simulink model "test_onoff_button_legitbehavior"  (R2022b)
settings: Solver=FixedStepAuto  StartTime=0.0  StopTime=240  FixedStep=0.1  RelTol=1e-3
settings Model: Creator=cristian  LastModifiedBy=cristian
settings ConfigComp: CovEnable=on  RecordCoverage=on  CovModelRefEnable=on

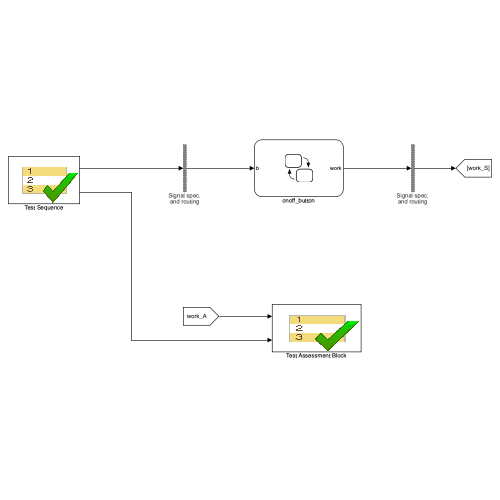
[thumbnail: Simulink's stored preview of the top-level diagram]
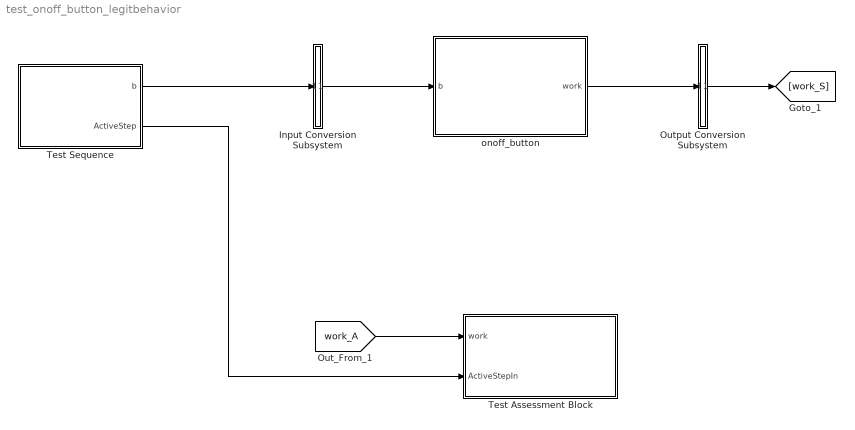
== system test_onoff_button_legitbehavior ==
  Input Conversion Subsystem : Subsystem  Tag=__SLT_ICS__  Description=|
      | Signal spec.
      | and routing
      settings: AttributesFormatString=%<Description>
  Output Conversion Subsystem : Subsystem  Tag=__SLT_OCS__  Description=|
      | Signal spec.
      | and routing
      settings: AttributesFormatString=%<Description>
  Test Assessment Block : Test Sequence  Tag=__SLT_ASMT__  TreatAsAtomicUnit=on
  Test Sequence : Test Sequence  TreatAsAtomicUnit=on
  onoff_button : Stateflow chart  TreatAsAtomicUnit=on
  wires:
  Output Conversion Subsystem/1(Outport_1) -> [work_S]
  Input Conversion Subsystem/1(Outport_1) -> onoff_button/1(b)
  onoff_button/1(work) -> Output Conversion Subsystem/1(Inport_1)
  Test Sequence/1(b) -> Input Conversion Subsystem/1(Inport_1)
  Test Sequence/2(ActiveStep) -> Test Assessment Block/2(ActiveStepIn)
  [work_A] -> Test Assessment Block/1(work)

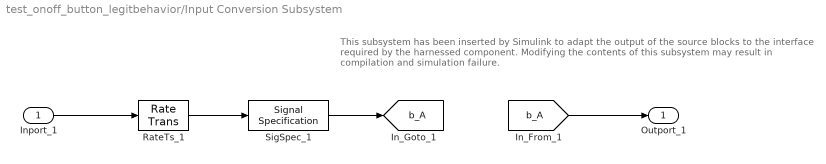
== system test_onoff_button_legitbehavior/Input Conversion Subsystem ==
  note: This subsystem has been inserted by Simulink to adapt the output of the source blocks to the interface required by the harnessed component.
      |  Modifying the contents of this subsystem may result in compilation and simulation failure.
  Inport_1 : Inport
  RateTs_1 : RateTransition  OutPortSampleTime=[-1, 0]
  SigSpec_1 : SignalSpecification  OutDataTypeStr=boolean  Dimensions=[1]  SampleTime=[-1, 0]
  Outport_1 : Outport
  tag scope: b_A=global
  wires:
  [b_A] -> Outport_1/1
  SigSpec_1/1 -> [b_A]
  RateTs_1/1 -> SigSpec_1/1
  Inport_1/1 -> RateTs_1/1

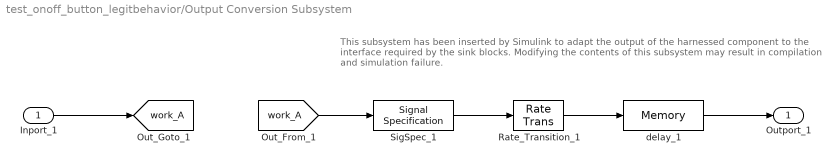
== system test_onoff_button_legitbehavior/Output Conversion Subsystem ==
  note: This subsystem has been inserted by Simulink to adapt the output of the harnessed component to the interface required by the sink blocks.
      |  Modifying the contents of this subsystem may result in compilation and simulation failure.
  Inport_1 : Inport
  Rate_Transition_1 : RateTransition  OutPortSampleTimeOpt=Inherit
  SigSpec_1 : SignalSpecification  OutDataTypeStr=boolean  Dimensions=[1]
  delay_1 : Memory
  Outport_1 : Outport
  tag scope: work_A=global
  wires:
  Inport_1/1 -> [work_A]
  [work_A] -> SigSpec_1/1
  SigSpec_1/1 -> Rate_Transition_1/1
  Rate_Transition_1/1 -> delay_1/1
  delay_1/1 -> Outport_1/1

== stateflow chart test_onoff_button_legitbehavior/Test Assessment Block ==
  state LegitBehavior
    state Run
      state Verify_LB_Init
        verify(work == 0);
      state Verify_LB_Press
        verify(work == 1);
      state Verify_CB_Release
        verify(work == 1);
      state Verify_LB_LongPress
        verify(work == 1);
      state Verify_LB_ReleaseLongPression
        verify(work == 0);
      state Verify_LB_Void
      (junction 388) -> (junction 391) [order 2]
      (junction 387) -> (junction 388) [order 1] : [ActiveStepIn == ActiveStepEnumH2.LB_Init
          | ]
      (junction 388) -> Verify_LB_Init [order 1] : [~in(LegitBehavior.Run.Verify_LB_Init)]
      (junction 94) -> Verify_LB_Press [order 1] : [~in(LegitBehavior.Run.Verify_LB_Press)]
      (junction 84) -> (junction 94) [order 1] : [ActiveStepIn == ActiveStepEnumH2.LB_Press
          | ]
      (junction 94) -> (junction 97) [order 2]
      (junction 84) -> (junction 101) [order 2]
      (junction 101) -> (junction 102) [order 1] : [ActiveStepIn == ActiveStepEnumH2.LB_Release
          | ]
      (junction 102) -> Verify_CB_Release [order 1] : [~in(LegitBehavior.Run.Verify_CB_Release)]
      (junction 101) -> (junction 356) [order 2]
      (junction 102) -> (junction 105) [order 2]
      (junction 356) -> (junction 357) [order 1] : [ActiveStepIn == ActiveStepEnumH2.LB_LongPress
          | ]
      (junction 357) -> Verify_LB_LongPress [order 1] : [~in(LegitBehavior.Run.Verify_LB_LongPress)]
      (junction 356) -> (junction 139) [order 2]
      (junction 357) -> (junction 360) [order 2]
      (junction 139) -> (junction 140) [order 1] : [ActiveStepIn == ActiveStepEnumH2.LB_ReleaseLongPression
          | ]
      (junction 140) -> Verify_LB_ReleaseLongPression [order 1] : [~in(LegitBehavior.Run.Verify_LB_ReleaseLongPression)]
      (junction 139) -> (junction 148) [order 2]
      (junction 140) -> (junction 143) [order 2]
      (junction 148) -> (junction 149)
      (junction 149) -> Verify_LB_Void [order 1] : [~in(LegitBehavior.Run.Verify_LB_Void)]
      (junction 149) -> (junction 152) [order 2]
      (junction 387) -> (junction 84) [order 2]
      Run -> (junction 387)
      (default) -> (junction 387)
    (default) -> Run
  (default) -> LegitBehavior : {assert(Active_Scenario_Index == 1,'The value of Scenario Parameter ''Active_Scenario_Index'' is not valid. Use the index of the scenario to specify it.')}
  data: work input boolean size=[1]; ActiveStepIn input; Active_Scenario_Index parameter =1

== stateflow chart test_onoff_button_legitbehavior/onoff_button ==
  note: Stato di accensione del bottone onoff
  note: In questo stato il bottone può accendere la macchina
  state INACTIVE
    state Pressed
      en: work = HIGH
    state Wait
      en: work = LOW
    (default) -> INACTIVE.Wait
    INACTIVE.Wait -> INACTIVE.Pressed : [b == PRESSED]
  note: Stato di spegnimento del bottone onoff
  note: In questo stato il bottone può spengere la macchina
  state ACTIVE
    state Wait
      en:
      b_long = RELEASED
    state Pressed
      en:
      b_long = RELEASED;
      on after(DURATION,sec): b_long = PRESSED
    state LongPressed
      en: work = LOW;
    (default) -> ACTIVE.Wait
    ACTIVE.Wait -> ACTIVE.Pressed : [b == PRESSED]
    ACTIVE.Pressed -> ACTIVE.Wait [order 1] : [b == RELEASED]
    ACTIVE.Pressed -> LongPressed [order 2] : [b_long == PRESSED && b == PRESSED]
  note: Se il bottone viene premuto una sola volta, il sistema viene acceso.
      | Se il bottone viene premuto per 1 secondo, il sistema viene spento.
      | Una pressione prolungata senza rilascio del bottone, non causa un alternarsi di accensioni e spegnimenti continui.
  (default) -> INACTIVE
  INACTIVE.Pressed -> ACTIVE : [b == RELEASED]
  LongPressed -> INACTIVE : [b==RELEASED]
  data: PRESSED constant boolean size=1 =0; RELEASED constant boolean size=1 =1; b input boolean size=1; DURATION constant double size=1 =1; b_long local boolean size=1; HIGH constant boolean size=1 =1; LOW constant boolean size=1 =0; work output boolean size=1

== stateflow chart test_onoff_button_legitbehavior/Test Sequence ==
  settings: updateMethod=DISCRETE  sampleTime=0.1
  state LegitBehavior
    state LB_Init
      b = true
    state LB_Press
      b = false
      settings: description=|
          | Il bottone viene premuto per la prima volta.
          | L'output in questo caso è alto alla singola pressione.
          | Indipendentemente dal tempo in cui permango, non dovrei cambiare stato.
    state LB_Release
      b = true
      settings: description=|
          | Il bottone viene rilasciato.
          | Il sistema dovrebbe prepararsi al comportamento di un bottone a livelli, quindi cambia stato.
    state LB_LongPress
      b = false
      settings: description=|
          | Pressione prolungata, dopo DURATION secondi (1, in questo caso) dovrei ottenere l'output in uscita.
          | Mi mantengo in pressione per il tempo necessario all'impostazione dell'output, più un sample time.
    state LB_ReleaseLongPression
      b = false
      settings: description=|
          | Rilascio il bottone dopo la pressione prolungata.
          | Il sistema dovrebbe preparasi al comportamento di un bottone semplice.
    state LB_Backto_Inactive
      b = true
    (default) -> LB_Init
    LB_Init -> LB_Press : [
        | true
        | ]
    LB_Press -> LB_Release : [
        | after(sample_time, sec)
        | ]
    LB_Release -> LB_LongPress : [
        | true
        | ]
    LB_LongPress -> LB_ReleaseLongPression : [
        | after(1+sample_time, sec)
        | ]
    LB_ReleaseLongPression -> LB_Backto_Inactive : [
        | true
        | ]
  (default) -> LegitBehavior : {assert(Active_Scenario_Index == 1,'The value of Scenario Parameter ''Active_Scenario_Index'' is not valid. Use the index of the scenario to specify it.')}
  data: b output boolean size=[1]; Active_Scenario_Index parameter =1; ActiveStep output Enum: ActiveStepEnumH2; sample_time constant double =str2num(get_param('InductionCooker','FixedStep'))
